simulink model "model_lab_2"  (R2021b)
settings: Solver=VariableStepAuto  StartTime=0.0  StopTime=1  RelTol=1e-3
model workspace (MAT data in the model file):
  U = 0
values from neighbouring files (symbols this model uses):
  J = 0.0024    [PControl.m]    (also in PIDControl.m; lab3-robotcar.m; lab3_on_off.m)
  Ke = 0.4870    (= 0.487)    [PControl.m]    (also in PIDControl.m; lab3-robotcar.m; lab3_on_off.m)
  Km = Ke    (= 0.487)    [PControl.m]    (also in PIDControl.m; lab3-robotcar.m; lab3_on_off.m)
  L = Ta * R    (= 0.000416420092144)    [PControl.m]    (also in PIDControl.m; lab3-robotcar.m; lab3_on_off.m = 0.0047)
  R = 8.8696    [PControl.m]    (also in PIDControl.m; lab3-robotcar.m; lab3_on_off.m)
settings Model: SimulationMode=accelerator  Creator=huynh  LastModifiedBy=huynh

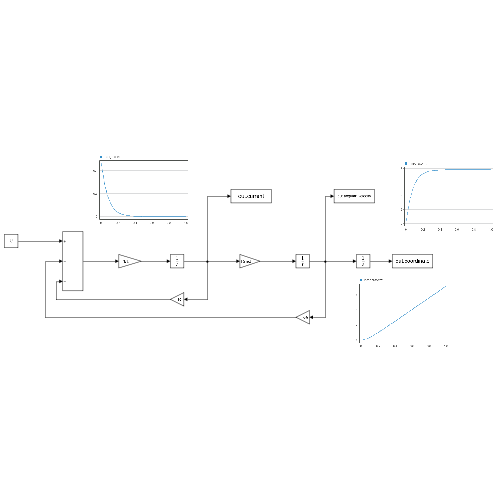
[thumbnail: Simulink's stored preview of the top-level diagram]
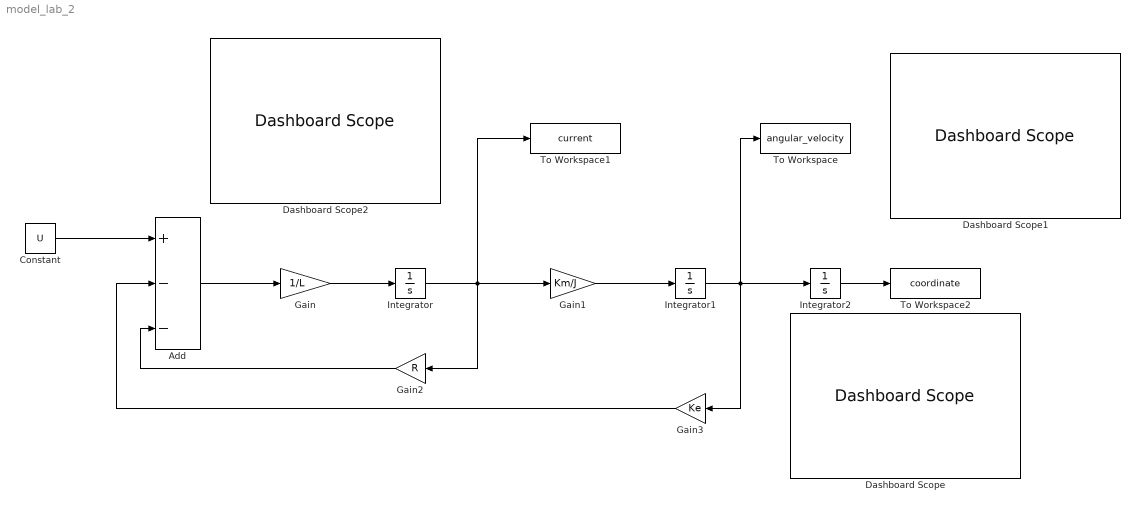
== system model_lab_2 ==
  Add : Sum  Inputs=+--
  Constant : Constant  Value=U
  Dashboard Scope : DashboardScope
  Dashboard Scope1 : DashboardScope
  Dashboard Scope2 : DashboardScope
  Gain : Gain  Gain=1/L
  Gain1 : Gain  Gain=Km/J
  Gain2 : Gain  Gain=R
  Gain3 : Gain  Gain=Ke
  Integrator : Integrator
  Integrator1 : Integrator
  Integrator2 : Integrator
  To Workspace : ToWorkspace  VariableName=angular_velocity  SaveFormat=Timeseries  SampleTime=-1
  To Workspace1 : ToWorkspace  VariableName=current  SaveFormat=Timeseries  SampleTime=-1
  To Workspace2 : ToWorkspace  VariableName=coordinate  SaveFormat=Timeseries  SampleTime=-1
  wires:
  Constant/1 -> Add/1
  Gain/1 -> Integrator/1
  Add/1 -> Gain/1
  Gain1/1 -> Integrator1/1
  Integrator1/1 -> Integrator2/1, Gain3/1, To Workspace/1
  Integrator/1 -> Gain2/1, To Workspace1/1, Gain1/1
  Gain2/1 -> Add/3
  Gain3/1 -> Add/2
  Integrator2/1 -> To Workspace2/1
